simulink library "ITKLib"  (R2022b)
settings: Solver=FixedStepDiscrete  StartTime=0.0  StopTime=10.0  FixedStep=0.01  RelTol=1e-3  EnableMultiTasking=on
values from neighbouring files (symbols this model uses):
  Glb_WhlRollgRd_SC = single(0.36)    [init_Global.m]
undefined symbols (not defined in the file or in its folder): docblock, SlDemoSign, SlDemoSign_Positive_SC, TaskTime_100ms_SC, TaskTime_10ms_SC, VehRefSpd_vMaxRefSpd_C
libraries: simulink x51, $bdroot x45, ITKLib_V14 x1
(part 2 of 10)

== system ITKLib/Filter ==
  GradientLimiter : Subsystem  RTWFcnName=GradientLimiter  RTWFileName=BoschITK_Mdl_Lib  mask(GradientLimiter){}
      mask help:
      | The output value is limited in its gradient to the last input value. The maximum valid difference is LU, the minimum valid difference is LD.
      | LD and LL have to be given with respect to sample time dT.
      |
      | inputs:
      | LU  - upper limit for gradient, LU≥0
      | LL  - lower limit for gradient，LL≤0
      | u   - signal to be evaluated
      | dT  - sample time for gradient calculation
      |
      | outputs:
      | y       - limited gradient
      |
      | Simulink Custom Model Library, created by MCC.
      settings: RTWFcnNameOpts=User specified  RTWFileNameOpts=User specified
      mask Display:
      | color('black');
      | plot([0.2,0.8],[0.5,0.5]);
      | plot([0.5,0.5],[0.2,0.8]);
      | plot([0.75,0.8,0.75],[0.53,0.5,0.47]);
      | plot([0.53,0.5,0.47],[0.75,0.8,0.75]);
      | color('red');
      | plot([0.2,0.3,0.7,0.8],[0.3,0.3,0.7,0.7]);
      | color('blue');
      | plot([0.6,0.66,0.63,0.6],[0.3,0.3,0.4,0.3]);
      | text(0.7,0.35,'/dT');
      | color('green');
      | text(1,0,'ITK','horizontalAlignment','right','verticalAlignment','bottom');
  GradientLimiterRRV : Subsystem  RTWFcnName=GradientLimiterRRV  RTWFileName=BoschITK_Mdl_Lib  mask(GradientLimiterRRV){}
      mask help:
      | The output value is limited in its gradient to the last input value. The maximum valid difference is LU, the minimum valid difference is LD.
      | LD and LL have to be given with respect to sample time dT.
      |
      | inputs:
      | LU  - upper limit for gradient, LU≥0
      | LL  - lower limit for gradient，LL≤0
      | u   - signal to be evaluated
      | E   - enable calculation
      | R   - reset block and forward RV to output signal
      | dT  - sample time for gradient calculation
      |
      | outputs:
      | y       - limited gradient
      |
      | Simulink Custom Model Library, created by MCC.
      settings: RTWFcnNameOpts=User specified  RTWFileNameOpts=User specified
      mask Display:
      | color('black');
      | plot([0.2,0.8],[0.5,0.5]);
      | plot([0.5,0.5],[0.2,0.8]);
      | plot([0.75,0.8,0.75],[0.53,0.5,0.47]);
      | plot([0.53,0.5,0.47],[0.75,0.8,0.75]);
      | color('blue');
      | plot([0.2,0.3,0.7,0.8],[0.3,0.3,0.7,0.7]);
      | plot([0.6,0.66,0.63,0.6],[0.3,0.3,0.4,0.3]);
      | text(0.7,0.35,'/dT');
      | color('green');
      | text(1,0,'ITK','horizontalAlignment','right','verticalAlignment','bottom');
  GrdtAtFlgChg : Subsystem  RTWFcnName=GrdtAtFlgChg  RTWFileName=MCC_Mdl_Lib  mask(GrdtAtFlgChg){}
      mask help:
      | Transition from the old value of u to new u based on Grdt when TransFlg changes.
      |
      | inputs:
      | u  - Input value
      | TransFlg   - transition flag
      | Grdt   - transition gradient
      | dT - sample time
      |
      | outputs:
      | TransOut - transition output
      | TransEnd - transition End flag
      | TransActv - transition active flag
      |
      | Simulink Custom Model Library, created by MCC.
      settings: MinAlgLoopOccurrences=on  RTWFcnNameOpts=User specified  RTWFileNameOpts=User specified
      mask Display:
      | color('green');
      | text(1,0,'ITK','horizontalAlignment','right','verticalAlignment','bottom');
  LowPass : Subsystem  RTWFcnName=LowPass  RTWFileName=BoschITK_Mdl_Lib  mask(LowPass){}
      mask help:
      | This block performs a first order lowpass filter with T as time constant, the relationship between the cut-off-frequency (f_c) and T:
      |
      |                                              (-f_c*dT*2*pi)
      |                         T  = dT/(1 - e                     )
      |
      |                          f_c  = -ln(dT/T-1)/(dT*2*pi)
      |
      | inputs:
      | T  - time constant
      | u   - signal to be evaluated
      | dT  - sample time
      |
      | outputs:
      | y       - signal after filtered
      |
      | Simulink Custom Model Library, created by MCC.
      settings: RTWFcnNameOpts=User specified  RTWFileNameOpts=User specified
      mask Display:
      | color('black');
      | port_label('output',1,'y');
      | port_label('input',1,'T');
      | port_label('input',2,'u');
      | port_label('input',3,'dT');
      | plot([0.2,0.8],[0.2,0.2]);
      | plot([0.2,0.2],[0.2,0.8]);
      | plot([0.2,0.3],[0.65,0.65]);
      | plot([0.35,0.45],[0.65,0.65]);
      | plot([0.5,0.6],[0.65,0.65]);
      | plot([0.65,0.75],[0.65,0.65]);
      | plot([0.75,0.8,0.75],[0.22,0.2,0.18]);
      | plot([0.18,0.2,0.22],[0.75,0.8,0.75])
      | color('red');
      | plot([0.2,0.3,0.4,0.5,0.6,0.7,0.8],[0.2,0.36,0.47,0.55,0.6,0.63,0.65]);
      | color('blue');
      | text(0.65,0.45,'T');
      | color('green');
      | text(1,0,'ITK','horizontalAlignment','right','verticalAlignment','bottom');
  LowPassERRV : Subsystem  RTWFcnName=LowPass_ERRV  RTWFileName=BoschITK_Mdl_Lib  mask(LowPassERRV){}
      mask help:
      | This block performs a first order lowpass filter with T as time constant, the relationship between the cut-off-frequency (f_c) and T:
      |
      |                                              (-f_c*dT*2*pi)
      |                         T  = dT/(1 - e                     )
      |
      |                          f_c  = -ln(dT/T-1)/(dT*2*pi)
      |
      | inputs:
      | T  - time constant
      | u   - signal to be evaluated
      | E   - enable calculation
      | R   - reset block and forward RV to output signal
      | dT  - sample time
      |
      | outputs:
      | y       - signal after filtered
      |
      | Simulink Custom Model Library, created by MCC.
      settings: RTWFcnNameOpts=User specified  RTWFileNameOpts=User specified
      mask Display:
      | color('orange');
      | port_label('input',3,'E');
      | port_label('input',4,'R');
      | color('black');
      | port_label('output',1,'y');
      | port_label('input',1,'T');
      | port_label('input',2,'u');
      | port_label('input',5,'RV');
      | port_label('input',6,'dT');
      | plot([0.2,0.8],[0.2,0.2]);
      | plot([0.2,0.2],[0.2,0.8]);
      | plot([0.2,0.3],[0.65,0.65]);
      | plot([0.35,0.45],[0.65,0.65]);
      | plot([0.5,0.6],[0.65,0.65]);
      | plot([0.65,0.75],[0.65,0.65]);
      | plot([0.75,0.8,0.75],[0.22,0.2,0.18]);
      | plot([0.18,0.2,0.22],[0.75,0.8,0.75])
      | color('blue');
      | plot([0.2,0.3,0.4,0.5,0.6,0.7,0.8],[0.2,0.36,0.47,0.55,0.6,0.63,0.65]);
      | text(0.65,0.45,'T');
      | color('green');
      | text(1,0,'ITK','horizontalAlignment','right','verticalAlignment','bottom');
  LowPassFrq : Subsystem  RTWFcnName=LowPass  RTWFileName=BoschITK_Mdl_Lib  mask(LowPassFrq){}
      mask help:
      | This block performs a first order lowpass filter with T as time constant, the relationship between the cut-off-frequency (f_c) and T:
      |
      |                                              (-f_c*dT*2*pi)
      |                         T  = dT/(1 - e                     )
      |
      |                          f_c  = -ln(dT/T-1)/(dT*2*pi)
      |
      | inputs:
      | u   - signal to be evaluated;
      | Frq  - frequency;
      | dT  - sample time;
      |
      | outputs:
      | y       - signal after filtered
      |
      | Simulink Custom Model Library, created by MCC.
      settings: RTWFcnNameOpts=User specified  RTWFileNameOpts=User specified
      mask Display:
      | color('black');
      | port_label('output',1,'y');
      | port_label('input',1,'u');
      | port_label('input',2,'Frq');
      | port_label('input',3,'dT');
      | plot([0.2,0.8],[0.2,0.2]);
      | plot([0.2,0.2],[0.2,0.8]);
      | plot([0.2,0.3],[0.65,0.65]);
      | plot([0.35,0.45],[0.65,0.65]);
      | plot([0.5,0.6],[0.65,0.65]);
      | plot([0.65,0.75],[0.65,0.65]);
      | plot([0.75,0.8,0.75],[0.22,0.2,0.18]);
      | plot([0.18,0.2,0.22],[0.75,0.8,0.75]);
      | color('red');
      | plot([0.2,0.3,0.4,0.5,0.6,0.7,0.8],[0.65,0.65,0.65,0.4,0.3,0.28,0.28]);
      | color('blue');
      | text(0.65,0.45,'Frq');
      | color('green');
      | text(1,0,'ITK','horizontalAlignment','right','verticalAlignment','bottom');
  LowPassFrqERRV : Subsystem  RTWFcnName=LowPass_ERRV  RTWFileName=BoschITK_Mdl_Lib  mask(LowPassERRV){}
      mask help:
      | This block performs a first order lowpass filter with T as time constant, the relationship between the cut-off-frequency (f_c) and T:
      |
      |                                              (-f_c*dT*2*pi)
      |                         T  = dT/(1 - e                     )
      |
      |                          f_c  = -ln(dT/T-1)/(dT*2*pi)
      |
      | inputs:
      | T  - time constant
      | u   - signal to be evaluated
      | E   - enable calculation
      | R   - reset block and forward RV to output signal
      | dT  - sample time
      |
      | outputs:
      | y       - signal after filtered
      |
      | Simulink Custom Model Library, created by MCC.
      settings: RTWFcnNameOpts=User specified  RTWFileNameOpts=User specified
      mask Display:
      | color('orange');
      | port_label('input',3,'E');
      | port_label('input',4,'R');
      | color('black');
      | port_label('output',1,'y');
      | port_label('input',1,'u');
      | port_label('input',2,'Frq');
      | port_label('input',5,'RV');
      | plot([0.2,0.8],[0.2,0.2]);
      | plot([0.2,0.2],[0.2,0.8]);
      | plot([0.2,0.3],[0.65,0.65]);
      | plot([0.35,0.45],[0.65,0.65]);
      | plot([0.5,0.6],[0.65,0.65]);
      | plot([0.65,0.75],[0.65,0.65]);
      | plot([0.75,0.8,0.75],[0.22,0.2,0.18]);
      | plot([0.18,0.2,0.22],[0.75,0.8,0.75])
      | color('blue');
      | plot([0.2,0.3,0.4,0.5,0.6,0.7,0.8],[0.2,0.36,0.47,0.55,0.6,0.63,0.65]);
      | text(0.65,0.45,'T');
      | color('green');
      | text(1,0,'ITK','horizontalAlignment','right','verticalAlignment','bottom');
  MoveAvrgFilt : Subsystem  RTWFcnName=MoveAvrgFilt  RTWFileName=MCC_Mdl_Lib  mask(MoveAvrgFilt){}
      mask help: Simulink Custom Model Library, created by MCC.
      settings: MinAlgLoopOccurrences=on  RTWFcnNameOpts=User specified  RTWFileNameOpts=User specified
      mask Display:
      | % color('black');
      | % plot([0.2,0.8],[0.5,0.5]);
      | % plot([0.5,0.5],[0.2,0.8]);
      | % plot([0.75,0.8,0.75],[0.53,0.5,0.47]);
      | % plot([0.53,0.5,0.47],[0.75,0.8,0.75]);
      | % color('blue');
      | % plot([0.2,0.3,0.7,0.8],[0.3,0.3,0.7,0.7]);
      | % plot([0.6,0.66,0.63,0.6],[0.3,0.3,0.4,0.3]);
      | % text(0.7,0.35,'/dT');
      | color('green');
      | text(1,0,'ITK','horizontalAlignment','right','verticalAlignment','bottom');
  MovgMinMaxAvrg : Stateflow chart  TreatAsAtomicUnit=on  mask(MovgMinMaxAvrg){}
      mask help:
      | The module calculates the minimum maximum average of the input signal's cyclic movement over a certain period of time.
      | Input signals:
      |             In: input signal, single data type;
      |             DataNr: cyclic counter value, uint16 data type;
      |
      | Output signals:
      |             Min: the minimum value of In, single data type;
      |             Max: the maximum value of In, single data type;
      |             Avrg: the average value of In, single data type;
      | the dimension of InBufAry is [1 DataNr].
      | For example, if DataNr = 10.
      | at step 11, Min is the minimum value of input in 1 through 11, and Max is the maximum value of input in 1 through 11, Avrg is the average value of input in 1 through 11;
      | at step 12, Min  is the minimum value of input in 2 through 12, and Max is the maximum value of input in 2 through 12, Avrg is the average value of input in 2 through 12;
      | at step 19, Min is the minimum value of input in 9 through 19, and Max is the maximum value of input in 9 through 19, Avrg is the average value of input in 9 through 19;
      | at step 20, Min is the minimum value of input in 10 through 20, Max is the maximum value of input in 10 through 20, Avrg is the average value of input in 10 through 20;
      |
      | Simulink Custom Model Library, created by MCC.
  RampLimiter : Subsystem  RTWFcnName=GradientLimiterRRV  RTWFileName=BoschITK_Mdl_Lib  mask(RampLimiter){}
      mask help:
      | Limit Up Function:
      | Input(k) > Output(k-1)，if Input(k) – Output(k-1) ≤ LimitUp，Output(k) = Input(k)，else Output(k) = Output(k-1) + LimitUp
      | Limit Down Function:
      | Input(k) < Output(k-1)，if Output(k-1) - Input(k) ≤ LimitDown，Output(k) = Input(k)，else Output(k) = Output(k-1) - LimitDown
      | The function is enabled only when Enable = 1
      settings: RTWFcnNameOpts=User specified  RTWFileNameOpts=User specified
      mask Display:
      | color('black');
      | plot([0.2,0.8],[0.5,0.5]);
      | plot([0.5,0.5],[0.2,0.8]);
      | plot([0.75,0.8,0.75],[0.53,0.5,0.47]);
      | plot([0.53,0.5,0.47],[0.75,0.8,0.75]);
      | color('red');
      | plot([0.2,0.3,0.7,0.8],[0.3,0.3,0.7,0.7]);
      | color('blue');
      | plot([0.6,0.66,0.63,0.6],[0.3,0.3,0.4,0.3]);
      | text(0.7,0.35,'/dT');
      | color('green');
      | text(1,0,'ITK','horizontalAlignment','right','verticalAlignment','bottom');
  RampTran : Subsystem  RTWFcnName=RampTrans  RTWFileName=MCC_Mdl_Lib  mask(RampTran){}
      mask help:
      | Transfer from IniVal to TarVar during T time when Ena is actived
      |
      | inputs:
      | IniVal  - Initial value of transition, single signal;
      | TarVal  - Target value of transition, single signal;
      | Type   - Transition type(int8 signal, 0:Linear line, 1:Convex line, -1:Concave line)
      | T   - Value transfer time, single signal, unit → s;
      | Ena   - Active transfer when equal to 1, otherwise reset to InitVal, boolean signal;
      | dT - sample time for mean calculation, single signal, unit → s;
      |
      | outputs:
      | Out - Ramp transition output value, single signal;
      | End - Ramp transition end flag, boolean signal;
      | TransActv - Ramp transition active flag, boolean signal;
      |
      | Simulink Custom Model Library, created by MCC.
      settings: RTWFcnNameOpts=User specified  RTWFileNameOpts=User specified
      mask Display:
      | color('black')
      | port_label('input', 1, 'T', 'texmode', 'on')
      | port_label('input', 2, 'IniVal', 'texmode', 'on')
      | port_label('input', 3, 'TarVal', 'texmode', 'on')
      | color('blue')
      | port_label('input', 4, 'Type', 'texmode', 'on')
      | color('orange')
      | port_label('input', 5, 'Ena', 'texmode', 'on')
      | color('black')
      | port_label('input', 6, 'dT', 'texmode', 'on')
      | port_label('output', 1, 'Out', 'texmode', 'on')
      | color('orange')
      | port_label('output', 2, 'End', 'texmode', 'on')
      | color('green')
      | port_label('output', 3, 'TranActv', 'texmode', 'on')
      | 
      | color('blue');
      | plot([0.2,0.3,0.4,0.5,0.6,0.7,0.8],[0.2,0.2,0.35,0.5,0.65,0.8,0.8]);
      | text(0.5,0.56,'0');
      | color('orange');
      | plot([0.2,0.3,0.4,0.5,0.6,0.7,0.8],[0.2,0.2,0.68,0.75,0.78,0.8,0.8]);
      | text(0.45,0.75,'1');
      | color('red');
      | plot([0.2,0.3,0.4,0.5,0.6,0.7,0.8],[0.2,0.2,0.22,0.25,0.32,0.8,0.8]);
      | text(0.55,0.25,'-1');
  SRampTran : Subsystem  RTWFcnName=SRampTrans  RTWFileName=JaevRI_Mdl_Lib  mask(SCurveRampTran){}
      mask help:
      | Transfer from IniVal to TarVar during T time when Ena is actived
      |
      | inputs:
      | IniVal  - Initial value of transition, single signal;
      | TarVal  - Target value of transition, single signal;
      | Type   - Transition type(int8 signal, 0:Convex prior S line, 1:Concave prior S line)
      | T   - Value transfer time, single signal, unit → s;
      | Ena   - Active transfer when equal to 1, otherwise reset to InitVal, boolean signal;
      | dT - sample time for mean calculation, single signal, unit → s;
      |
      | outputs:
      | Out - S Ramp transition output value, single signal;
      | End - S Ramp transition end flag, boolean signal;
      | TransActv - S Ramp transition active flag, boolean signal;
      |
      | Simulink Custom Model Library, created by MCC.
      settings: RTWFcnNameOpts=User specified  RTWFileNameOpts=User specified
      mask Display:
      | color('black')
      | port_label('input', 1, 'T', 'texmode', 'on')
      | port_label('input', 2, 'IniVal', 'texmode', 'on')
      | port_label('input', 3, 'TarVal', 'texmode', 'on')
      | color('blue')
      | port_label('input', 4, 'Type', 'texmode', 'on')
      | color('orange')
      | port_label('input', 5, 'Ena', 'texmode', 'on')
      | color('black')
      | port_label('input', 6, 'dT', 'texmode', 'on')
      | port_label('output', 1, 'Out', 'texmode', 'on')
      | color('orange')
      | port_label('output', 2, 'End', 'texmode', 'on')
      | color('green')
      | port_label('output', 3, 'TranActv', 'texmode', 'on')
      | 
      | color('orange');
      | plot([0.2,0.25,0.3,0.35,0.4,0.45,0.5,0.55,0.6,0.65,0.7,0.75,0.8],[0.2,0.2,0.45,0.47,0.48,0.49,0.5,0.51,0.52,0.53,0.55,0.8,0.8]);
      | text(0.3,0.5,'0');
      | color('red');
      | plot([0.2,0.25,0.3,0.35,0.4,0.45,0.5,0.55,0.6,0.65,0.7,0.75,0.8],[0.2,0.2,0.21,0.22,0.23,0.25,0.5,0.75,0.77,0.78,0.79,0.8,0.8]);
      | text(0.5,0.25,'1');
  SecOrdBPF : Subsystem  RTWFcnName=LowPass  RTWFileName=BoschITK_Mdl_Lib  mask(SecOrdBPF){}
      mask help:
      | This block performs a second order bandpass filter .
      | inputs:
      | u   - signal to be evaluated ;
      | Frq  - frequency;
      | dT  - sample time;
      | Zeta -damping ratio;
      |
      | outputs:
      | y       - signal after filtered
      settings: RTWFcnNameOpts=User specified  RTWFileNameOpts=User specified
      mask Display:
      | color('black');
      | port_label('output',1,'y');
      | port_label('input',1,'u');
      | port_label('input',2,'Frq');
      | port_label('input',3,'Zeta');
      | port_label('input',4,'dT');
      | plot([0.2,0.8],[0.2,0.2]);
      | plot([0.2,0.2],[0.2,0.8]);
      | plot([0.2,0.3],[0.65,0.65]);
      | plot([0.35,0.45],[0.65,0.65]);
      | plot([0.5,0.6],[0.65,0.65]);
      | plot([0.65,0.75],[0.65,0.65]);
      | plot([0.75,0.8,0.75],[0.22,0.2,0.18]);
      | plot([0.18,0.2,0.22],[0.75,0.8,0.75])
      | color('red');
      | plot([0.2,0.35,0.4,0.45,0.5,0.55,0.6,0.65,0.8],[0.28,0.3,0.35,0.65,0.65,0.65,0.35,0.3,0.28]);
      | color('blue');
      | text(0.65,0.45,'Frq');
      | color('green');
      | text(1,0,'ITK','horizontalAlignment','right','verticalAlignment','bottom');

== system ITKLib/Hysteresis ==
  HysteresisA : Subsystem  Description=HysteresisA  RTWFcnName=HysteresisA  RTWFileName=BoschITK_Mdl_Lib  mask(HysteresisA){}
      mask help:
      | (R > L)
      | If u ≥ R output becomes 1,
      | If u ≤ L output becomes 0,
      | otherwise the output stays the same (InitialValue false)
      |
      | Simulink Custom Model Library, created by MCC.
      settings: AttributesFormatString=%<Description>  MinAlgLoopOccurrences=on  RTWFcnNameOpts=User specified  RTWFileNameOpts=User specified
      mask Help:
      | If u > R output becomes 1,
      | If u < L unterschritten output becomes 0,
      | otherwise the output stays the same (InitialValue false)
      mask Display:
      | color('black');
      | port_label('output',1,'A');
      | color('black');
      | port_label('input',1,'R');
      | port_label('input',2,'u');
      | port_label('input',3,'L');
      | color('red');
      | plot([0.2 0.8],[0.1,0.1]);
      | plot([0.3 0.9],[0.6,0.6]);
      | plot([0.3 0.3],[0.1,0.6]);
      | plot([0.8 0.8],[0.1,0.6]);
      | plot([0.25 0.3],[0.4 0.3]);
      | plot([0.3 0.35],[0.3 0.4]);
      | plot([0.75 0.8],[0.3 0.4]);
      | plot([0.8 0.85],[0.4 0.3]);
      | color('blue');
      | text(0.3,0.78,'L');
      | text(0.75,0.78,'R');
      | color('green');
      | text(1,0,'ITK','horizontalAlignment','right','verticalAlignment','bottom');
  HysteresisB : Subsystem  Description=HysteresisB  RTWFcnName=HysteresisB  RTWFileName=BoschITK_Mdl_Lib  mask(HysteresisB){}
      mask help:
      | (R > L)
      | If u ≥ R output becomes 0,
      | If u ≤ L output becomes 1,
      | otherwise the output stays the same (InitialValue false)
      |
      | Simulink Custom Model Library, created by MCC.
      settings: AttributesFormatString=%<Description>  RTWFcnNameOpts=User specified  RTWFileNameOpts=User specified
      mask Help:
      | If u > R output becomes 0,
      | If u < L unterschritten output becomes 1,
      | otherwise the output stays the same (InitialValue false)
      mask Display:
      | color('black');
      | port_label('output',1,'B');
      | color('black');
      | port_label('input',1,'R');
      | port_label('input',2,'u');
      | port_label('input',3,'L');
      | color('red');
      | plot([0.2 0.8],[0.1,0.1]);
      | plot([0.3 0.9],[0.6,0.6]);
      | plot([0.3 0.3],[0.1,0.6]);
      | plot([0.8 0.8],[0.1,0.6]);
      | plot([0.25 0.3],[0.3 0.4]);
      | plot([0.3 0.35],[0.4 0.3]);
      | plot([0.75 0.8],[0.4 0.3]);
      | plot([0.8 0.85],[0.3 0.4]);
      | color('blue');
      | text(0.3,0.78,'L');
      | text(0.75,0.78,'R');
      | color('green');
      | text(1,0,'ITK','horizontalAlignment','right','verticalAlignment','bottom');

== system ITKLib/Limit ==
  Limit : Subsystem  Description=""  RTWFcnName=Limit  RTWFileName=BoschITK_Mdl_Lib  mask(LimitWoFlag){}
      mask help:
      | Limits the input value u between the maximum (MX) and the minimum (MN) values.
      |
      | The input value u is checked first against the minimum value and then against the maximum value.
      |
      | In addition to that a flag is set in case the current value is higher than MX and another flag is set in case the current value is smaller than the MN value.
      |
      | inputs:
      | MX  - maximum allowed value
      | MN  - minimal allowed value
      | u   - input value to be evaluated
      |
      | outputs:
      | y       - limited output value
      |
      | Simulink Custom Model Library, created by MCC.
      settings: RTWFcnNameOpts=User specified  RTWFileNameOpts=User specified
      mask Display:
      | color('black');
      | plot([0.2,0.8],[0.5,0.5]);
      | plot([0.5,0.5],[0.2,0.8]);
      | plot([0.75,0.8,0.75],[0.53,0.5,0.47]);
      | plot([0.53,0.5,0.47],[0.75,0.8,0.75]);
      | color('red');
      | plot([0.2,0.3,0.7,0.8],[0.3,0.3,0.7,0.7]);
      | color('green');
      | text(1,0,'ITK','horizontalAlignment','right','verticalAlignment','bottom');
  LimitAndExcess : Subsystem  Description=""  RTWFcnName=LimitAndExcess  RTWFileName=BoschITK_Mdl_Lib  mask(LimitAndExcess){}
      mask help:
      | Limits the input value u between the maximum (MX) and the minimum (MN) values.
      |
      | The input value u is checked first against the minimum value and then against the maximum value.
      |
      |
      | inputs:
      | MX  - maximum allowed value;
      | MN  - minimal allowed value;
      | u   - input value to be evaluated;
      |
      | outputs:
      | y       - limited output value;
      | ExceUpLim   -  if input value is higher than MX, ExceUpLim = u - MX;
      | ExceLowLim 	- if input value is less than MN, ExceUpLim = u - MN
      |
      | Simulink Custom Model Library, created by MCC.
      settings: RTWFcnNameOpts=User specified  RTWFileNameOpts=User specified
      mask Display:
      | color('black');
      | plot([0.2,0.7],[0.5,0.5]);
      | plot([0.45,0.45],[0.2,0.8]);
      | plot([0.65,0.7,0.65],[0.53,0.5,0.47]);
      | plot([0.43,0.45,0.48],[0.75,0.8,0.75]);
      | color('red');
      | plot([0.2,0.3,0.6,0.7],[0.3,0.3,0.7,0.7]);
      | color('green');
      | text(1,0,'ITK','horizontalAlignment','right','verticalAlignment','bottom');
  LimitAndFlag : Subsystem  Description=""  RTWFcnName=LimitAndFlag  RTWFileName=BoschITK_Mdl_Lib  mask(LimitWFlag){}
      mask help:
      | Limits the input value u between the maximum (MX) and the minimum (MN) values.
      |
      | The input value u is checked first against the minimum value and then against the maximum value.
      |
      | In addition to that a flag is set in case the current value is higher than MX and another flag is set in case the current value is smaller than the MN value.
      |
      | inputs:
      | MX  - maximum allowed value
      | MN  - minimal allowed value
      | u   - input value to be evaluated
      |
      | outputs:
      | y             - limited output value
      | bMax      - true, if input value is higher than MX
      | bMin       - true, if input value is less than MN
      | LimFlag   - true, if input value is less than MN or higher than MX
      |
      | Simulink Custom Model Library, created by MCC.
      settings: RTWFcnNameOpts=User specified  RTWFileNameOpts=User specified
      mask Display:
      | color('black');
      | plot([0.2,0.7],[0.5,0.5]);
      | plot([0.45,0.45],[0.2,0.8]);
      | plot([0.65,0.7,0.65],[0.53,0.5,0.47]);
      | plot([0.43,0.45,0.48],[0.75,0.8,0.75]);
      | color('red');
      | plot([0.2,0.3,0.6,0.7],[0.3,0.3,0.7,0.7]);
      | color('green');
      | text(1,0,'ITK','horizontalAlignment','right','verticalAlignment','bottom');
  LimitOnly : Subsystem  Description=""  RTWFcnName=Limit  RTWFileName=BoschITK_Mdl_Lib  mask(LimitOnly){}
      mask help:
      | Limits the input value u between the maximum (Max) and the minimum (Min) values.
      |
      | inputs:
      | Max  - maximum allowed value
      | Min  - minimal allowed value
      | u   - input value to be evaluated
      |
      | outputs:
      | y       - limited output value
      |
      | Simulink Custom Model Library, created by MCC.
      settings: RTWFcnNameOpts=User specified  RTWFileNameOpts=User specified
      mask Display:
      | color('black');
      | plot([0.2,0.8],[0.5,0.5]);
      | plot([0.5,0.5],[0.2,0.8]);
      | plot([0.75,0.8,0.75],[0.53,0.5,0.47]);
      | plot([0.53,0.5,0.47],[0.75,0.8,0.75]);
      | color('red');
      | plot([0.2,0.3,0.7,0.8],[0.3,0.3,0.7,0.7]);
      | color('green');
      | text(1,0,'ITK','horizontalAlignment','right','verticalAlignment','bottom');
      | color('blue');
      | text(0.7,0.85,'LimOnly','horizontalAlignment','right','verticalAlignment','bottom');
  Saturation2 : Saturate  UpperLimit=10  LowerLimit=0
      settings: AttributesFormatString=|
      | UpperLimit = %<UpperLimit>
      | LowLimit = %<LowerLimit>
  UpdFac : Subsystem  mask(UpdFac){}
      mask help:
      | Update the factor and status.
      |
      | inputs:
      | NewFac  - New factor value, single data type, the maximum value is 1,the minimum value is 0;
      | OldFac  - Old factor value, the maximum value is 1,the minimum value is 0;
      | NewFacSt  - The status of new factor value, uint8 data type;
      | OldFacSt  - The status of old factor value, uint8 data type;
      |
      | outputs:
      | Fac      - The output factor value, single data type, the maximum value is 1,the minimum value is 0; if NewFac is lower than OldFac, then Fac is NewFac, otherwise Fac is OldFac;
      | FacSt      - The status of factor value, single data type, the maximum value is 1,the minimum value is 0; if NewFac is lower than OldFac, then FacSt is NewFacSt, otherwise FacSt is OldFacSt;
      |
      | Simulink Custom Model Library, created by MCC.
  UpdMaxMin : Subsystem  mask(UpdMaxMin){}
      mask help:
      | Update the maximum and minimum value, the status of  the maximum and minimum value.
      |
      | inputs:
      | NewMax  - New maximum value;
      | OldMax  - Old maximum value;
      | NewMaxSt  - The status of new maximum value;
      | OldMaxSt  - The status of old maximum value;
      | NewMin  - New minimum value;
      | OldMin  - Old minimum value;
      | NewMinSt  - The status of new minimum value;
      | OldMinSt  - The status of old minimum value;
      |
      | outputs:
      | Max      - The maximum value, if NewMax is lower than OldMax, then Max is NewMax, otherwise Max is OldMax;
      | MaxSt      - The status of maximum value, if NewMax is lower than OldMax, then MaxSt is NewMaxSt, otherwise MaxSt is OldMaxSt;
      | Min      - The minimum value, if NewMin is upper than OldMin, then Min is NewMin, otherwise Mrin is OldMin;
      | MinSt      - The status of minimum value, if NewMin is upper than OldMin, then MinSt is NewMinSt, otherwise Mrin is OldMinSt;
      |
      | Simulink Custom Model Library, created by MCC.

== system ITKLib/Memory ==
  EdgeBi : Subsystem  Tag=initial value = 0  RTWFcnName=EdgeBi  RTWFileName=ITK_Mdl_Lib  mask(EdgeBi){}
      mask help:
      | Detects a rising or falling edge on the input signal.
      |
      | The initial value the input signal is compared to during the first execution step needs to be specified within mask.
      |
      | INPUT:
      | u               - input signal (boolean)
      | Initial Value   - value for first comparison (mask value)
      |
      | OUTPUTS:
      | y - output bit > set when input bit changes
      |
      | Simulink Custom Model Library, created by MCC.
      mask init:
      | pos = get_param(gcb, 'Position');
      | x_c = (pos(3) - pos(1))/2;
      | y_c = (pos(4) - pos(2))/2;
      | y_c1 = y_c+5;
      | y_c2 = y_c-5;
      | sc1 = 10;
      | sc2 = 12;
      | sc3 = 4;
      | sc4 = 3;
      | sc5 = 3;
      settings: RTWFcnNameOpts=User specified  RTWFileNameOpts=User specified
      mask Display:
      | color('blue');
      | plot([x_c-sc1,x_c,x_c,x_c+sc1],[y_c-sc2,y_c-sc2,y_c+sc2,y_c+sc2]);
      | plot([x_c-sc3,x_c,x_c+sc3],[y_c1-sc4,y_c1+sc5,y_c1-sc4]);
      | plot([x_c-sc3,x_c,x_c+sc3],[y_c2+sc4,y_c2-sc5,y_c2+sc4]);
  EdgeFalling : Subsystem  Tag=initial value = 0  RTWFcnName=EdgeFalling  RTWFileName=ITK_Mdl_Lib  mask(EdgeFalling){}
      mask help:
      | Detects a falling edge on the input signal.
      |
      | The initial value the input signal is compared to during the first execution step is "false".
      |
      | INPUT:
      | u - input signal (boolean)
      |
      | OUTPUTS:
      | y - output bit > set when input bit changes from 1 - 0
      |
      | Simulink Custom Model Library, created by MCC.
      mask init:
      | pos = get_param(gcb, 'Position');
      | x_c = (pos(3) - pos(1))/2;
      | y_c = (pos(4) - pos(2))/2;
      | sc1 = 8;
      | sc2 = 8;
      | sc3 = 4;
      | sc4 = 3;
      | sc5 = 3;
      settings: RTWFcnNameOpts=User specified  RTWFileNameOpts=User specified
      mask Display:
      | color('blue');
      | plot([x_c-sc1,x_c,x_c,x_c+sc1],[y_c+sc2,y_c+sc2,y_c-sc2,y_c-sc2]);
      | plot([x_c-sc3,x_c,x_c+sc3],[y_c+sc4,y_c-sc5,y_c+sc4]);
  EdgeRising : Subsystem  Tag=initial value = 0  RTWFcnName=EdgeRising  RTWFileName=ITK_Mdl_Lib  mask(EdgeRising){}
      mask help:
      | Detects a rising edge on the input signal.
      |
      | The initial value the input signal is compared to during the first execution step is "false".
      |
      | INPUT:
      | u - input signal (boolean)
      |
      | OUTPUTS:
      | y - output bit > set when input bit changes from 0 - 1
      |
      | Simulink Custom Model Library, created by MCC.
      mask init:
      | pos = get_param(gcb, 'Position');
      | x_c = (pos(3) - pos(1))/2;
      | y_c = (pos(4) - pos(2))/2;
      | sc1 = 8;
      | sc2 = 8;
      | sc3 = 4;
      | sc4 = 3;
      | sc5 = 3;
      mask Display:
      | color('blue');
      | plot([x_c-sc1,x_c,x_c,x_c+sc1],[y_c-sc2,y_c-sc2,y_c+sc2,y_c+sc2]);
      | plot([x_c-sc3,x_c,x_c+sc3],[y_c-sc4,y_c+sc5,y_c-sc4]);
      | % color('green');
      | % text(1,0,'ITK','horizontalAlignment','right','verticalAlignment','bottom');
  RSLatch : Subsystem  RTWFcnName=RS_Latch  RTWFileName=ITK_Mdl_Lib  mask(RSLatch){}
      mask help:
      | RS latch with initial value
      | Set signal is passed from port 'S'
      | Reset signal is passed from port 'R'
      | Initial value is passed from port 'IV'
      |
      | Q is set if S is set and reset if R is set.
      | The reset logic is of higher priority than set logic.
      | The initial state is set by IV.
      |
      | Simulink Custom Model Library, created by MCC.
      mask Help:
      | RS latch with initial value
      | Set signal is passed from port 'S'
      | Reset signal is passed from port 'R'
      | Initial value is passed from port 'IV'
      | 
      | Q is set if S is set and reset if R is set.
      | The reset logic is of higher priority than set logic.
      | The initial state is set by IV.
      mask Display:
      | color('blue')
      | disp('\fontsize{12}RS Latch', 'texmode', 'on')
      | color('black');
      | port_label('input', 1, 'S', 'texmode', 'on')
      | port_label('input', 2, 'R', 'texmode', 'on')
      | port_label('output', 1, 'Q', 'texmode', 'on')
      | color('green');
      | text(1,0,'ITK','horizontalAlignment','right','verticalAlignment','bottom');
  Unit Delay : UnitDelay  SampleTime=-1  HasFrameUpgradeWarning=on
      settings: AttributesFormatString=<initial=%<x0>>
  UnitDelay : UnitDelay  SampleTime=-1  HasFrameUpgradeWarning=on
      settings: AttributesFormatString=<Initial=%<x0>>

== system ITKLib/PID ==
  PIController : Subsystem  RTWFcnName=PIDControlLimited  RTWFileName=BoschITK_Mdl_Lib  mask(PIControl){}
      mask help:
      | PIControl
      | Input parameters：
      | Max: the maximum value of output y;
      | Min: the minimum value of output y;
      | u: the input control difference;
      | PreC: the feed forward value;
      | R: the reset flag of Ki;
      | RV: the reset value of Ki;
      | Simulink Custom Model Library, created by MCC.
      settings: RTWFcnNameOpts=User specified  RTWFileNameOpts=User specified
      mask Display:
      | color('blue')
      | fprintf('PI Controller');
      | color('green');
      | text(1,0,'ITK','horizontalAlignment','right','verticalAlignment','bottom');
  PICtrlrWithLimFlg : Subsystem  RTWFcnName=PIDControlLimited  RTWFileName=BoschITK_Mdl_Lib  mask(PICtrlrWithLimFlg){}
      mask help:
      | PIControl
      | Input parameters：
      | Max: the maximum value of output y;
      | Min: the minimum value of output y;
      | KpOutMax: the maximum value of Kp out;
      | KpOutMin: the minimum value of Kp out;
      | u: the input control difference;
      | PreC: the feed forward value;
      | R: the reset flag of Ki;
      | RV: the reset value of Ki;
      | Output parameters：
      | y: PI output value;
      | KiOut: Ki output value;
      | KpOut: Kp output value;
      | UpLimActv: when y >= Max, UpLimActv is true, otherwise  UpLimActv is false;
      | LoLimActv: when y <= Min, LoLimActv is true, otherwise  LoLimActv is false;
      |
      | Simulink Custom Model Library, created by MCC.
      settings: RTWFcnNameOpts=User specified  RTWFileNameOpts=User specified
      mask Display:
      | color('blue')
      | % fprintf('PI Controller With Limmit Flag');
      | % fprintf('PICtrlrWithLimFlg');
      | text(0.15,0.5, 'PICtrlrWithLimFlg');
      | color('green');
      | text(1,0,'ITK','horizontalAlignment','right','verticalAlignment','bottom');
  PIGovernor : Subsystem  mask(PIGovernor){}
      mask help:
      | u: the input control difference;
      | PreC: the feed forward value;
      | Max: the maximum value of output y;
      | Min: the minimum value of output y;
      | Ena: the enable flag of PI governor
      | R: the reset flag of Ki;
      | RV: the reset value of Ki;
      mask Display:
      | color('blue')
      | fprintf('PI Governor');
      | color('green');
      | text(1,0,'ITK','horizontalAlignment','right','verticalAlignment','bottom');

== system ITKLib/Special ==
  ControlAlgorithm : Subsystem
      mask Display:
      | color('green')
      | fprintf('ControlAlgorithm')
  Copyright : simulink/Model-Wide Utilities/Model Info  Frame=on  DisplayStringWithTags=|  HorizontalTextAlignment=Left  LeftAlignmentValue=0.02
      | © ITK Engineering Technology (Wu Xi) Co., Ltd. (ITKC)
      | 
      | Model Version: %<ModelVersion>
      | Date: %<LastModificationDate>
  Detailed Function Description : simulink/Model-Wide Utilities/DocBlock  Tag=HideFromReport  DocumentType=Text
      content=|
      | No detailed function description available!
  Diagramm Chapter : Subsystem  Tag=HideFromReport  InitFcn=docblock('save_document',gcb);  mask(DocBlock){ECoderFlag=, DocumentType=Text, PicFile=0}
      mask prompts: ECoderFlag "Simulink:masks:DocBlockEmbeddedCoderFlagLabel_MP"; DocumentType "Simulink:masks:DocBlockDocTypeLabel_MP"; PicFile "Picture File"
      mask help: Simulink:masks:DocBlock_MD
      settings: DeleteFcn=docblock('close_document',gcb);  PreSaveFcn=docblock('save_document',gcb);
      mask TypeOptions DocumentType: Simulink:masks:Text | Simulink:masks:RTF | Simulink:masks:HTML
      mask DialogControl ECoderFlag Prompt: 代码生成模板符号
      mask DialogControl DocumentType Prompt: 文档类型
      mask DialogControl BtnEditTxt Prompt: Edit Text
      mask DialogControl BtnEditTxt Callback: docblock('edit_document',gcb);
      mask DialogControl BtnLoadPic Prompt: Load Picture
      mask DialogControl BtnLoadPic Callback:
      | [file,filePath]=uigetfile('*.jpg;*.png','Select image...');
      | fprintf(1,'Selected %s%s\n',string(filePath),string(file));
      | try
      |     % Dummy: Check if file is valid picture
      |     Image = imread([filePath file]);
      |     set_param(gcb, 'PicFile', file);
      | 
      | catch
      |     fprintf(2,'No valid image selected!\n')
      | end
      mask Display:
      | % Add picture to center, with rotation settings "ON"
      | plot([.8 0 0 1 1 .8 .8 1],[1 1 0 0 .8 1 .8 .8]);
      | text(.5,.6,'DOC','horizontalalignment','center');
      | text(.9,.015,'Image','verticalalignment','bottom','horizontalalignment','right');
  Document : Subsystem
      mask Display:
      | color('green')
      | fprintf('Model\nDocument')
  HideInReport : Subsystem  Tag=HideFromReport  Description=This Block hides the system and the included subsystems from the report generation.  mask(HideFromReport){}
      mask help: This Block hides the system and the included subsystems from the report generation.
      mask Help: This Block hides the system and the included subsystems from the report generation.
      mask Display:
      | ud = get_param(gcb,'UserData');
      | image(ud.Image);
  Hints for Application : simulink/Model-Wide Utilities/DocBlock  Tag=HideFromReport  DocumentType=Text
      content=|
      | No Hints for application available!
  InlineDescription : Subsystem  Tag=HideFromReport  Description=Refer Detailed Function Description for detailed information.  mask(InlineDescription){ShowInLibBrowser=0, RefreshPar=0}
      mask help:
      | This block has an input dialog, which is written in the description of the parent Subsystem and the block description.
      | Before the model is saved, the description of the block is written in the description of the parent subsystem.
      mask Help:
      | This block has an input dialog, which is written in the description of the parent Subsystem and the block description.
      | Before the model is saved, the description of the block is written in the description of the parent subsystem.
      mask Display:
      | Description=get_param(gcs,'Description');
      | text(0.02,0.5,Description,'horizontalAlignment','left','verticalAlignment','middle');
  ReportWithParent : Subsystem  Tag=HideFromReport  Description=Effects that the subsystem is shown in the context of the parent subsystem  TreatAsAtomicUnit=on  mask{Parameter1=0}
      mask prompts: Parameter1 "HideMyPortToLib"
      mask Display:
      | s = ['Report',char(10),'With',char(10),'Parent'];
      | disp(s);
  RequirementDocumentation : Subsystem  Tag=HideFromReport  Description=Refer Detailed Function Description for detailed information.  mask(REQ_DOC){ReqId=REQ_DOC_DUMMY, ReqLink=LinkToRequirementSpecification}
      mask prompts: ReqId "Requirement Id"; ReqLink "Requirement Link"
      settings: DeleteFcn=InlineDescriptionCbHandler('DeleteFcn')
      mask DialogControl ReqOpenBtn Prompt: Open Link
      mask DialogControl ReqOpenBtn Callback:
      | reqLink = get_param(gcb,'ReqLink');
      | 
      | if(exist(reqLink,'file'))
      |     [filepath,name,ext] = fileparts(reqLink)
      |     set_param(gcb, 'ReqLink',  [name, ext]);
      |     open(reqLink);
      | else
      |     web(reqLink);
      | end;
      mask Display:
      | Description=get_param(gcb,'ReqId');
      | 
      | % Add an Icon from UserData to Block
      | % Get UserData
      | ud = get_param(gcb,'UserData');
      | % Add picture to center, with rotation settings "ON"
      | image(ud.Image,[.02, .02, .20 ,1.0],'on');
      | text(0.25,0.5,Description,'horizontalAlignment','left','verticalAlignment','middle');
  Revision History : Subsystem  Description=Subsystem to store the Revision History  mask(RevTable){ECoderFlag=, DocumentType=Text, revId=---, revVersion=---, revAuthor=---, revDate=-1, RevChanges=---, revTableDummy=0}
      mask prompts: ECoderFlag "Simulink:masks:DocBlockEmbeddedCoderFlagLabel_MP"; DocumentType "Simulink:masks:DocBlockDocTypeLabel_MP"; revId "Revision ID"; revVersion "Version"; revAuthor "Author"; revDate "Date"; RevChanges "Changes"
      mask help:
      | This block generates a revision table in its User data.
      |
      | If the "Date" field is set to -1, the block will automatically add the current date (YYYY-MM-DD)
      mask Help:
      | This block generates a revision table in its User data.
      | 
      | If the "Date" field is set to -1, the block will automatically add the current date (YYYY-MM-DD)
      mask TypeOptions DocumentType: Simulink:masks:Text | Simulink:masks:RTF | Simulink:masks:HTML
      mask DialogControl ECoderFlag Prompt: 代码生成模板符号
      mask DialogControl DocumentType Prompt: 文档类型
      mask DialogControl Control2 Prompt: Edit Document
      mask DialogControl Control2 Callback: docblock('edit_document',gcb);
      mask DialogControl Container4 Prompt: Controls
      mask DialogControl Control4 Prompt: Add Rev. Entry
      mask DialogControl Control4 Callback: revTableBlockHandler(gcbh,'addEntry');
      mask DialogControl Control6 Prompt: Open Rev. Table in WS
      mask DialogControl Control6 Callback: revTableBlockHandler(gcbh,'paste2Ws')
      mask DialogControl Container3 Prompt: Revision History
      mask Display:
      | plot([.8 0 0 1 1 .8 .8 1],[1 1 0 0 .8 1 .8 .8]);
      | text(.5,.6,'REV','horizontalalignment','center');
      | %text(.95,.05,get_param(gcb,'DocumentType'),'verticalalignment','bottom','horizontalalignment','right');
  Scope : Scope
